simulink model "planemodel"  (Simulink 8.6)
settings: Solver=ode15s  SolverMode=SingleTasking  StartTime=0.0  StopTime=10  MaxStep=0.1  RelTol=1e-3  AbsTol=1e-3
values from neighbouring files (symbols this model uses):
  A = [ -1.3936    0.9744   -0.0019   -0.5349   -0.0071   -1.0562    0.4891 ... (first row only)    [jasdata.m]
  B = [ 0     0 ... (first row only)    [jasdata.m]
  C = [ 1     0     0     0     0     0     0 ... (first row only)    [jasdata.m]
  D = [ 0     0 ... (first row only)    [jasdata.m]
  Kf = 0.4*[1 1]    [design1.m]    (also in design2.m = 1.27*[1 1]; design3.m = 1.27*[1 1])
  T_f = 0.3    [design1.m]    (also in design2.m; design3.m = 0.03; sol5.m = 0.03)
undefined symbols (not defined in the file): Ctheta, L
libraries: pilotlib x1
settings Model: Creator=sven  LastModifiedBy=dell  ExtModeTrigMode=oneshot  ExtModeArmWhenConnect=off
settings DataIOCC: LimitDataPoints=off  SaveOutput=off  SaveTime=off
settings OptimizationCC: BlockReduction=off  BooleanDataType=off  ExpressionDepthLimit=128
settings DebuggingCC: SaveWithParameterizedLinksMsg=none  SignalResolutionControl=TryResolveAllWithWarning  SolverPrmCheckMsg=none  MultiTaskDSMMsg=warning  MultiTaskCondExecSysMsg=none  FcnCallInpInsideContextMsg=EnableAllAsError  StateNameClashWarn=none
settings HardwareCC: ProdBitPerPointer=64  ProdLargestAtomicFloat=Float  ProdIntDivRoundTo=Zero  ProdEndianess=LittleEndian  ProdWordSize=64  ProdHWDeviceType=Intel->x86-64 (Windows64)  TargetUnknown=on
settings RTWCC: TemplateMakefile=grt_unix.tmf
settings GRTTargetCC: GeneratePreprocessorConditionals=Use local settings
settings ConfigComp: CovModelRefEnable=off

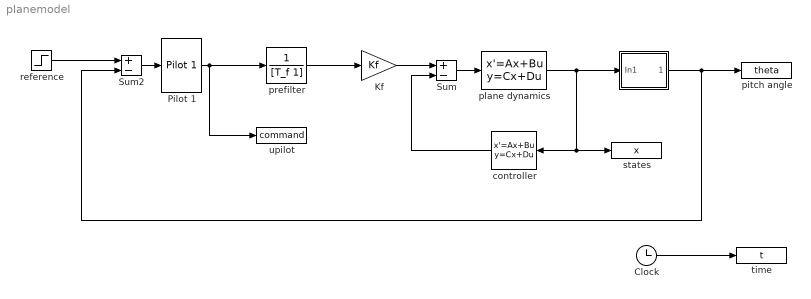
== system planemodel ==
  " " : Subsystem  mask(Matrix Gain){K=Ctheta}
      mask prompts: K "Gain matrix:"
      mask help: Matrix Gain.
      mask Help: Multiplies input vector by entered matrix to produce output vector (y=Au).
      mask Display: disp('Ctheta')
  Clock : Clock
  Kf : Gain  Gain=Kf  SaturateOnIntegerOverflow=on  OutDataTypeStr=Inherit: Same as input  ParamDataTypeStr=Inherit: Same as input
  Pilot 1 : pilotlib/Pilot 1
  Sum : Sum  Inputs=+-  SaturateOnIntegerOverflow=on  InputSameDT=on  OutDataTypeStr=Inherit: Same as first input
  Sum2 : Sum  Inputs=+-  SaturateOnIntegerOverflow=on  InputSameDT=on  OutDataTypeStr=Inherit: Same as first input
  controller : StateSpace  A=[]  B=[]  C=[]  D=K  X0=0  mask(Matrix gain){K=L}
      mask prompts: K "Gain matrix:"
      mask help: Matrix Gain:
      mask Help: Multiplies input vector by entered matrix to produce output vector.
      mask Display: disp('L')
  pitch angle : ToWorkspace  VariableName=theta
      settings: MaxDataPoints=10000
  plane dynamics : StateSpace  A=A  B=B  C=C  D=D  X0=0
  prefilter : TransferFcn  Denominator=[T_f 1]
  reference : Step  Time=0  SampleTime=0
  states : ToWorkspace  VariableName=x
      settings: MaxDataPoints=10000
  time : ToWorkspace  VariableName=t
      settings: MaxDataPoints=10000
  upilot : ToWorkspace  VariableName=command
      settings: MaxDataPoints=10000
  wires:
  " "/1(Out1) -> Sum2/2, pitch angle/1
  reference/1 -> Sum2/1
  plane dynamics/1 -> " "/1(In1), controller/1, states/1
  prefilter/1 -> Kf/1
  Sum/1 -> plane dynamics/1
  controller/1 -> Sum/2
  Kf/1 -> Sum/1
  Clock/1 -> time/1
  Sum2/1 -> Pilot 1/1
  Pilot 1/1 -> prefilter/1, upilot/1

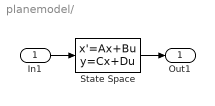
== system planemodel/  ==
  In1 : Inport
  State Space : StateSpace  A=[]  B=[]  C=[]  D=K  X0=0
  Out1 : Outport
  wires:
  In1/1 -> State Space/1
  State Space/1 -> Out1/1
